simulink model "lab1_simulink"  (R2016a)
settings: Solver=VariableStepAuto  StartTime=0.0  StopTime=10.0  MaxStep=0.001  RelTol=1e-3
settings Model: Creator=Karim  LastModifiedBy=Karim

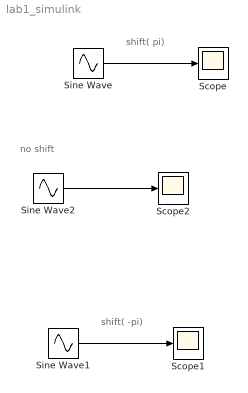
== system lab1_simulink ==
  note: no shift
  note: shift( pi)
  note: shift( -pi)
  Scope : Scope
  Scope1 : Scope
  Scope2 : Scope
  Sine Wave : Sin  Amplitude=10  Frequency=10*pi  Phase=pi  SampleTime=0
  Sine Wave1 : Sin  Amplitude=10  Frequency=10*pi  Phase=-pi  SampleTime=0
  Sine Wave2 : Sin  Amplitude=10  Frequency=10*pi  SampleTime=0
  wires:
  Sine Wave/1 -> Scope/1
  Sine Wave2/1 -> Scope2/1
  Sine Wave1/1 -> Scope1/1
